simulink model "SecRwLtStFwdBkwdTrgtPosSelc"  (R2018b)
settings: Solver=FixedStepDiscrete  StartTime=0.0  StopTime=10.0  FixedStep=0.01  RelTol=1e-3
undefined symbols (not defined in the file or in its folder): KeSMSw4SAcsMd21SecRwLtStFrwdBkwdPos_Val, KeSMSw4SAcsMd21SecRwLtStFrwdBkwdPosMax_Val, KeSMSw4SAcsMd21SecRwLtStFrwdBkwdPosMin_Val, KeSMSw4SAcsMd22SecRwLtStFrwdBkwdPos_Val, KeSMSw4SAcsMd22SecRwLtStFrwdBkwdPosMax_Val, KeSMSw4SAcsMd22SecRwLtStFrwdBkwdPosMin_Val, KeSMSw4SAcsMd25SecRwLtStFrwdBkwdPos_Val, KeSMSw4SAcsMd25SecRwLtStFrwdBkwdPosMax_Val, KeSMSw4SAcsMd25SecRwLtStFrwdBkwdPosMin_Val, KeSMSw4SAcsMd26SecRwLtStFrwdBkwdPos_Val, KeSMSw4SAcsMd26SecRwLtStFrwdBkwdPosMax_Val, KeSMSw4SAcsMd26SecRwLtStFrwdBkwdPosMin_Val, KeSMSw4SLegrstOpenMdSecRwLtStFrwdBkwdPos_Val, KeSMSw4SLegrstOpenMdSecRwLtStFrwdBkwdPosMax_Val, KeSMSw4SLegrstOpenMdSecRwLtStFrwdBkwdPosMin_Val, KeSMSw4SLyingMDSecRwLtStFrwdBkwdPos_Val, KeSMSw4SLyingMDSecRwLtStFrwdBkwdPosMax_Val, KeSMSw4SLyingMDSecRwLtStFrwdBkwdPosMin_Val, KeSMSw4SVIPMDSecRwLtStFrwdBkwdPos_Val, KeSMSw4SVIPMDSecRwLtStFrwdBkwdPosMax_Val, KeSMSw4SVIPMDSecRwLtStFrwdBkwdPosMin_Val, KeSMSw6sAcsEntrySecRwLtStFrwdBkwdPos_Val, KeSMSw6sAcsEntrySecRwLtStFrwdBkwdPosMax_Val, KeSMSw6sAcsEntrySecRwLtStFrwdBkwdPosMin_Val, KeSMSw6sAcsExtSecRwLtStFrwdBkwdPos_Val, KeSMSw6sAcsExtSecRwLtStFrwdBkwdPosMax_Val, KeSMSw6sAcsExtSecRwLtStFrwdBkwdPosMin_Val, KeSMSw6sFamilyMdSecRwLtStFrwdBkwdPos_Val, KeSMSw6sFamilyMdSecRwLtStFrwdBkwdPosMax_Val, KeSMSw6sFamilyMdSecRwLtStFrwdBkwdPosMin_Val, KeSMSw6sFamilyRMdSecRwLtStFrwdBkwdPos_Val, KeSMSw6sFamilyRMdSecRwLtStFrwdBkwdPosMax_Val, KeSMSw6sFamilyRMdSecRwLtStFrwdBkwdPosMin_Val, KeSMSw6sVIPSecRwLtStFrwdBkwdPos_Val, KeSMSw6sVIPSecRwLtStFrwdBkwdPosMax_Val, KeSMSw6sVIPSecRwLtStFrwdBkwdPosMin_Val, KeSMSwAcsEntrySecRwLtStFrwdBkwdPos_Val, KeSMSwAcsEntrySecRwLtStFrwdBkwdPosMax_Val, KeSMSwAcsEntrySecRwLtStFrwdBkwdPosMin_Val, KeSMSwAcsExtSecRwLtStFrwdBkwdPos_Val, KeSMSwAcsExtSecRwLtStFrwdBkwdPosMax_Val, KeSMSwAcsExtSecRwLtStFrwdBkwdPosMin_Val, KeSMSwAcsMd8SecRwLtStFrwdBkwdPos_Val, KeSMSwAcsMd8SecRwLtStFrwdBkwdPosMax_Val, KeSMSwAcsMd8SecRwLtStFrwdBkwdPosMin_Val, KeSMSwFamilyMdSecRwLtStFrwdBkwdPos_Val, KeSMSwFamilyMdSecRwLtStFrwdBkwdPosMax_Val, KeSMSwFamilyMdSecRwLtStFrwdBkwdPosMin_Val, KeSMSwFamilyRMdSecRwLtStFrwdBkwdPos_Val, KeSMSwFamilyRMdSecRwLtStFrwdBkwdPosMax_Val, KeSMSwFamilyRMdSecRwLtStFrwdBkwdPosMin_Val, KeSMSwVIPSecRwLtStFrwdBkwdPos_Val, KeSMSwVIPSecRwLtStFrwdBkwdPosMax_Val, KeSMSwVIPSecRwLtStFrwdBkwdPosMin_Val
libraries: TrgtPosSelcLib x15
settings Model: Creator=sn2xws  LastModifiedBy=sn2xws
settings Model: ModifiedHistory=|
  | 2023.8.1 V2.0.0 CR401790 增加模式21-26
  | 2023.11.16 V2.3.0 Issue 566045 全躺，vip，腿托打开增加前后位置
  | 2024.7.8 V3.0.0 557模式流程V1.9
settings DataIOCC: SaveFormat=StructureWithTime
settings OptimizationCC: DefaultParameterBehavior=Inlined  EnhancedBackFolding=on  PassReuseOutputArgsAs=Individual arguments  ZeroExternalMemoryAtStartup=off  ZeroInternalMemoryAtStartup=off  OptimizeBlockOrder=speed  DifferentSizesBufferReuse=on  OptimizationCustomize=off
settings DebuggingCC: ParameterTunabilityLossMsg=error
settings HardwareCC: ProdBitPerPointer=32  ProdBitPerSizeT=32  ProdBitPerPtrDiffT=32  ProdLargestAtomicFloat=None  ProdWordSize=32  ProdHWDeviceType=Renesas->RH850
settings ModelReferenceCC: ModelReferenceNumInstancesAllowed=Single
settings SFSimCC: MATLABDynamicMemAlloc=off
settings RTWCC: SystemTargetFile=autosar.tlc  GenCodeOnly=on  TemplateMakefile=ert_default_tmf  Description=AUTOSAR  GenerateReport=on  IncludeHyperlinkInReport=on  LaunchReport=on  GenerateTraceInfo=on  GenerateTraceReport=on  GenerateTraceReportSl=on  GenerateTraceReportSf=on  GenerateTraceReportEml=on  GenerateCodeMetricsReport=on
settings CodeAppCC: ForceParamTrailComments=on  IgnoreCustomStorageClasses=off  OperatorAnnotations=on  SimulinkDataObjDesc=on  SFDataObjDesc=on  InsertBlockDesc=on
settings STFCustomTargetCC: TargetLangStandard=C99 (ISO)  MultiwordLength=256  ParMdlRefBuildCompliant=on  CompOptLevelCompliant=on  IncludeMdlTerminateFcn=off  CombineOutputUpdateFcns=on  SuppressErrorStatus=on  ERTCustomFileBanners=on  SupportNonFinite=off  SupportComplex=off  SupportContinuousTime=off  SupportNonInlinedSFcns=off  RemoveResetFunc=on  MATLABClassNameForMDSCustomization=Simulink.SoftwareTarget.ERTCustomization  AutosarCompliant=on  UseToolchainInfoCompliant=on  LookupTableObjectStructAxisOrder=2,1,3,4,...  LUTObjectStructOrderEvenSpacing=Size,Table,Breakpoints  SystemTargetFile=autosar.tlc
settings ERTTargetCC: TargetLangStandard=C99 (ISO)  ConcurrentExecutionCompliant=off  IncludeMdlTerminateFcn=off  SuppressErrorStatus=on  SupportNonFinite=off  SupportComplex=off  ModelStepFunctionPrototypeControlCompliant=off  CPPClassGenCompliant=off  AutosarCompliant=on  LookupTableObjectStructAxisOrder=2,1,3,4,...  LUTObjectStructOrderEvenSpacing=Size,Table,Breakpoints  InlinedParameterPlacement=NonHierarchical  ERTCustomFileTemplate=example_file_process.tlc  ERTFilePackagingFormat=Compact

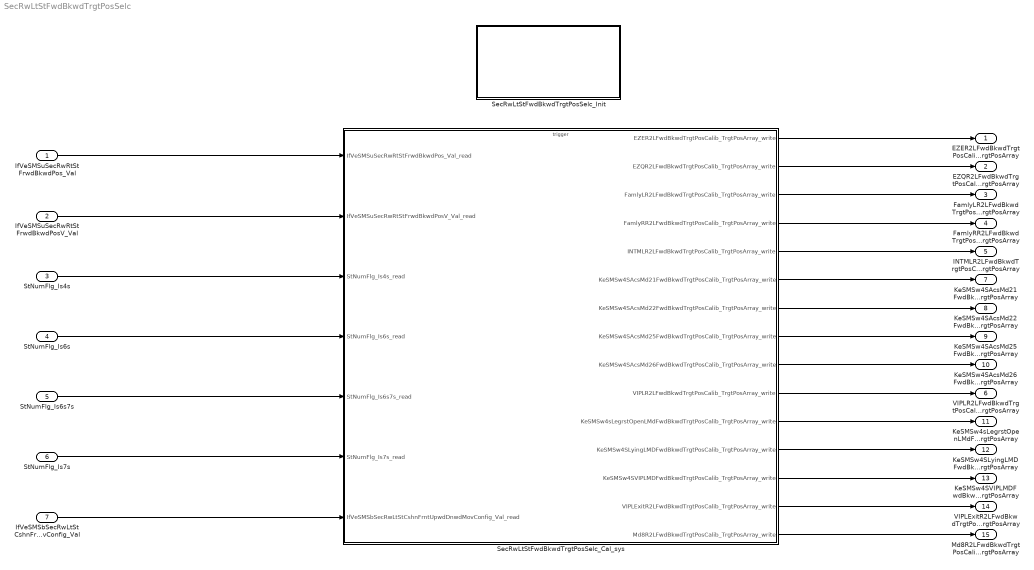
== system SecRwLtStFwdBkwdTrgtPosSelc ==
  IfVeSMSuSecRwRtStFrwdBkwdPos_Val : Inport  OutDataTypeStr=uint16  PortDimensions=1
  IfVeSMSuSecRwRtStFrwdBkwdPosV_Val : Inport  Port=2  OutDataTypeStr=boolean  PortDimensions=1
  StNumFlg_Is4s : Inport  Port=3  OutDataTypeStr=boolean  PortDimensions=1
  StNumFlg_Is6s : Inport  Port=4  OutDataTypeStr=boolean  PortDimensions=1
  StNumFlg_Is6s7s : Inport  Port=5  OutDataTypeStr=boolean  PortDimensions=1
  StNumFlg_Is7s : Inport  Port=6  OutDataTypeStr=boolean  PortDimensions=1
  IfVeSMSbSecRwLtStCshnFrntUpwdDnwdMovConfig_Val : Inport  Port=7  OutDataTypeStr=boolean  PortDimensions=1
  SecRwLtStFwdBkwdTrgtPosSelc_Cal_sys : Subsystem
  SecRwLtStFwdBkwdTrgtPosSelc_Init : Subsystem
  EZER2LFwdBkwdTrgtPosCalib_TrgtPosArray : Outport  Description=|  OutDataTypeStr=uint16  PortDimensions=3
      | 0:Pos
      | 1:Max
      | 2:Min
  EZQR2LFwdBkwdTrgtPosCalib_TrgtPosArray : Outport  Description=|  Port=2  OutDataTypeStr=uint16  PortDimensions=3
      | 0:Pos
      | 1:Max
      | 2:Min
  FamlyLR2LFwdBkwdTrgtPosCalib_TrgtPosArray : Outport  Description=|  Port=3  OutDataTypeStr=uint16  PortDimensions=3
      | 0:Pos
      | 1:Max
      | 2:Min
  FamlyRR2LFwdBkwdTrgtPosCalib_TrgtPosArray : Outport  Description=|  Port=4  OutDataTypeStr=uint16  PortDimensions=3
      | 0:Pos
      | 1:Max
      | 2:Min
  INTMLR2LFwdBkwdTrgtPosCalib_TrgtPosArray : Outport  Description=|  Port=5  OutDataTypeStr=uint16  PortDimensions=3
      | 0:Pos
      | 1:Max
      | 2:Min
  VIPLR2LFwdBkwdTrgtPosCalib_TrgtPosArray : Outport  Description=|  Port=6  OutDataTypeStr=uint16  PortDimensions=3
      | 0:Pos
      | 1:Max
      | 2:Min
  KeSMSw4SAcsMd21FwdBkwdTrgtPosCalib_TrgtPosArray : Outport  Description=|  Port=7  OutDataTypeStr=uint16  PortDimensions=3
      | 0:Pos
      | 1:Max
      | 2:Min
  KeSMSw4SAcsMd22FwdBkwdTrgtPosCalib_TrgtPosArray : Outport  Description=|  Port=8  OutDataTypeStr=uint16  PortDimensions=3
      | 0:Pos
      | 1:Max
      | 2:Min
  KeSMSw4SAcsMd25FwdBkwdTrgtPosCalib_TrgtPosArray : Outport  Description=|  Port=9  OutDataTypeStr=uint16  PortDimensions=3
      | 0:Pos
      | 1:Max
      | 2:Min
  KeSMSw4SAcsMd26FwdBkwdTrgtPosCalib_TrgtPosArray : Outport  Description=|  Port=10  OutDataTypeStr=uint16  PortDimensions=3
      | 0:Pos
      | 1:Max
      | 2:Min
  KeSMSw4sLegrstOpenLMdFwdBkwdTrgtPosCalib_TrgtPosArray : Outport  Description=|  Port=11  OutDataTypeStr=uint16  PortDimensions=3
      | 0:Pos
      | 1:Max
      | 2:Min
  KeSMSw4SLyingLMDFwdBkwdTrgtPosCalib_TrgtPosArray : Outport  Description=|  Port=12  OutDataTypeStr=uint16  PortDimensions=3
      | 0:Pos
      | 1:Max
      | 2:Min
  KeSMSw4SVIPLMDFwdBkwdTrgtPosCalib_TrgtPosArray : Outport  Description=|  Port=13  OutDataTypeStr=uint16  PortDimensions=3
      | 0:Pos
      | 1:Max
      | 2:Min
  VIPLExitR2LFwdBkwdTrgtPosCalib_TrgtPosArray : Outport  Description=|  Port=14  OutDataTypeStr=uint16  PortDimensions=3
      | 0:Pos
      | 1:Max
      | 2:Min
  Md8R2LFwdBkwdTrgtPosCalib_TrgtPosArray : Outport  Description=|  Port=15  OutDataTypeStr=uint16  PortDimensions=3
      | 0:Pos
      | 1:Max
      | 2:Min
  wires:
  IfVeSMSuSecRwRtStFrwdBkwdPos_Val/1 -> SecRwLtStFwdBkwdTrgtPosSelc_Cal_sys/1(IfVeSMSuSecRwRtStFrwdBkwdPos_Val_read)
  IfVeSMSuSecRwRtStFrwdBkwdPosV_Val/1 -> SecRwLtStFwdBkwdTrgtPosSelc_Cal_sys/2(IfVeSMSuSecRwRtStFrwdBkwdPosV_Val_read)
  StNumFlg_Is4s/1 -> SecRwLtStFwdBkwdTrgtPosSelc_Cal_sys/3(StNumFlg_Is4s_read)
  StNumFlg_Is6s/1 -> SecRwLtStFwdBkwdTrgtPosSelc_Cal_sys/4(StNumFlg_Is6s_read)
  StNumFlg_Is6s7s/1 -> SecRwLtStFwdBkwdTrgtPosSelc_Cal_sys/5(StNumFlg_Is6s7s_read)
  StNumFlg_Is7s/1 -> SecRwLtStFwdBkwdTrgtPosSelc_Cal_sys/6(StNumFlg_Is7s_read)
  SecRwLtStFwdBkwdTrgtPosSelc_Cal_sys/1(EZER2LFwdBkwdTrgtPosCalib_TrgtPosArray_write) -> EZER2LFwdBkwdTrgtPosCalib_TrgtPosArray/1
  SecRwLtStFwdBkwdTrgtPosSelc_Cal_sys/2(EZQR2LFwdBkwdTrgtPosCalib_TrgtPosArray_write) -> EZQR2LFwdBkwdTrgtPosCalib_TrgtPosArray/1
  SecRwLtStFwdBkwdTrgtPosSelc_Cal_sys/3(FamlyLR2LFwdBkwdTrgtPosCalib_TrgtPosArray_write) -> FamlyLR2LFwdBkwdTrgtPosCalib_TrgtPosArray/1
  SecRwLtStFwdBkwdTrgtPosSelc_Cal_sys/4(FamlyRR2LFwdBkwdTrgtPosCalib_TrgtPosArray_write) -> FamlyRR2LFwdBkwdTrgtPosCalib_TrgtPosArray/1
  SecRwLtStFwdBkwdTrgtPosSelc_Cal_sys/5(INTMLR2LFwdBkwdTrgtPosCalib_TrgtPosArray_write) -> INTMLR2LFwdBkwdTrgtPosCalib_TrgtPosArray/1
  SecRwLtStFwdBkwdTrgtPosSelc_Cal_sys/10(VIPLR2LFwdBkwdTrgtPosCalib_TrgtPosArray_write) -> VIPLR2LFwdBkwdTrgtPosCalib_TrgtPosArray/1
  SecRwLtStFwdBkwdTrgtPosSelc_Cal_sys/6(KeSMSw4SAcsMd21FwdBkwdTrgtPosCalib_TrgtPosArray_write) -> KeSMSw4SAcsMd21FwdBkwdTrgtPosCalib_TrgtPosArray/1
  SecRwLtStFwdBkwdTrgtPosSelc_Cal_sys/7(KeSMSw4SAcsMd22FwdBkwdTrgtPosCalib_TrgtPosArray_write) -> KeSMSw4SAcsMd22FwdBkwdTrgtPosCalib_TrgtPosArray/1
  SecRwLtStFwdBkwdTrgtPosSelc_Cal_sys/8(KeSMSw4SAcsMd25FwdBkwdTrgtPosCalib_TrgtPosArray_write) -> KeSMSw4SAcsMd25FwdBkwdTrgtPosCalib_TrgtPosArray/1
  SecRwLtStFwdBkwdTrgtPosSelc_Cal_sys/9(KeSMSw4SAcsMd26FwdBkwdTrgtPosCalib_TrgtPosArray_write) -> KeSMSw4SAcsMd26FwdBkwdTrgtPosCalib_TrgtPosArray/1
  SecRwLtStFwdBkwdTrgtPosSelc_Cal_sys/11(KeSMSw4sLegrstOpenLMdFwdBkwdTrgtPosCalib_TrgtPosArray_write) -> KeSMSw4sLegrstOpenLMdFwdBkwdTrgtPosCalib_TrgtPosArray/1
  SecRwLtStFwdBkwdTrgtPosSelc_Cal_sys/12(KeSMSw4SLyingLMDFwdBkwdTrgtPosCalib_TrgtPosArray_write) -> KeSMSw4SLyingLMDFwdBkwdTrgtPosCalib_TrgtPosArray/1
  SecRwLtStFwdBkwdTrgtPosSelc_Cal_sys/13(KeSMSw4SVIPLMDFwdBkwdTrgtPosCalib_TrgtPosArray_write) -> KeSMSw4SVIPLMDFwdBkwdTrgtPosCalib_TrgtPosArray/1
  IfVeSMSbSecRwLtStCshnFrntUpwdDnwdMovConfig_Val/1 -> SecRwLtStFwdBkwdTrgtPosSelc_Cal_sys/7(IfVeSMSbSecRwLtStCshnFrntUpwdDnwdMovConfig_Val_read)
  SecRwLtStFwdBkwdTrgtPosSelc_Cal_sys/14(VIPLExitR2LFwdBkwdTrgtPosCalib_TrgtPosArray_write) -> VIPLExitR2LFwdBkwdTrgtPosCalib_TrgtPosArray/1
  SecRwLtStFwdBkwdTrgtPosSelc_Cal_sys/15(Md8R2LFwdBkwdTrgtPosCalib_TrgtPosArray_write) -> Md8R2LFwdBkwdTrgtPosCalib_TrgtPosArray/1

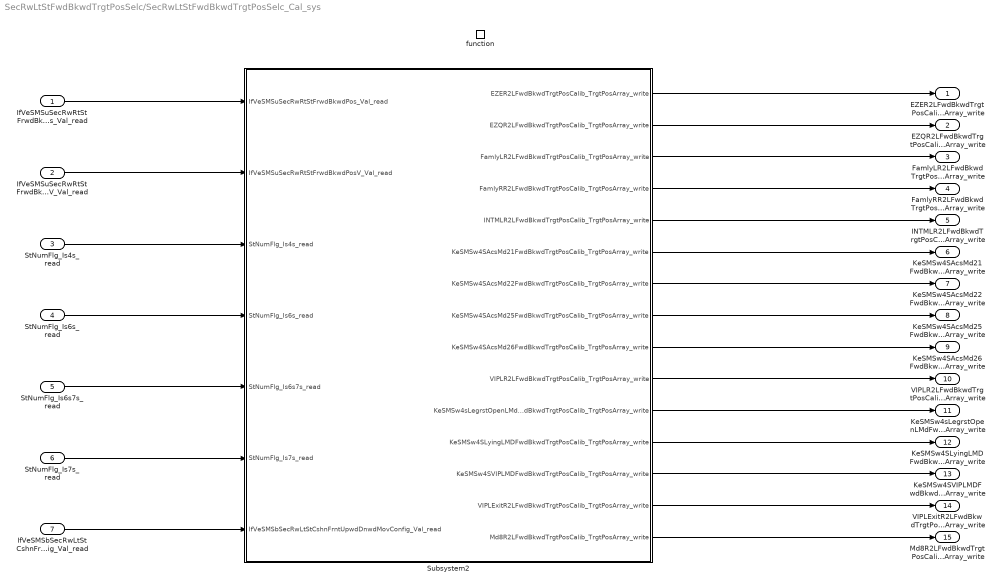
== system SecRwLtStFwdBkwdTrgtPosSelc/SecRwLtStFwdBkwdTrgtPosSelc_Cal_sys ==
  IfVeSMSuSecRwRtStFrwdBkwdPos_Val_read : Inport
  IfVeSMSuSecRwRtStFrwdBkwdPosV_Val_read : Inport  Port=2
  StNumFlg_Is4s_read : Inport  Port=3
  StNumFlg_Is6s_read : Inport  Port=4
  StNumFlg_Is6s7s_read : Inport  Port=5
  StNumFlg_Is7s_read : Inport  Port=6
  IfVeSMSbSecRwLtStCshnFrntUpwdDnwdMovConfig_Val_read : Inport  Port=7
  function : TriggerPort  TriggerType=function-call  IsSimulinkFunction=on  FunctionName=SecRwLtStFwdBkwdTrgtPosSelc_Cal  VariantControl=(inherit)
  Subsystem2 : Subsystem
  EZER2LFwdBkwdTrgtPosCalib_TrgtPosArray_write : Outport
      settings: EnsureOutportIsVirtual=on
  EZQR2LFwdBkwdTrgtPosCalib_TrgtPosArray_write : Outport  Port=2
      settings: EnsureOutportIsVirtual=on
  FamlyLR2LFwdBkwdTrgtPosCalib_TrgtPosArray_write : Outport  Port=3
      settings: EnsureOutportIsVirtual=on
  FamlyRR2LFwdBkwdTrgtPosCalib_TrgtPosArray_write : Outport  Port=4
      settings: EnsureOutportIsVirtual=on
  INTMLR2LFwdBkwdTrgtPosCalib_TrgtPosArray_write : Outport  Port=5
      settings: EnsureOutportIsVirtual=on
  KeSMSw4SAcsMd21FwdBkwdTrgtPosCalib_TrgtPosArray_write : Outport  Port=6
      settings: EnsureOutportIsVirtual=on
  KeSMSw4SAcsMd22FwdBkwdTrgtPosCalib_TrgtPosArray_write : Outport  Port=7
      settings: EnsureOutportIsVirtual=on
  KeSMSw4SAcsMd25FwdBkwdTrgtPosCalib_TrgtPosArray_write : Outport  Port=8
      settings: EnsureOutportIsVirtual=on
  KeSMSw4SAcsMd26FwdBkwdTrgtPosCalib_TrgtPosArray_write : Outport  Port=9
      settings: EnsureOutportIsVirtual=on
  VIPLR2LFwdBkwdTrgtPosCalib_TrgtPosArray_write : Outport  Port=10
      settings: EnsureOutportIsVirtual=on
  KeSMSw4sLegrstOpenLMdFwdBkwdTrgtPosCalib_TrgtPosArray_write : Outport  Port=11
      settings: EnsureOutportIsVirtual=on
  KeSMSw4SLyingLMDFwdBkwdTrgtPosCalib_TrgtPosArray_write : Outport  Port=12
      settings: EnsureOutportIsVirtual=on
  KeSMSw4SVIPLMDFwdBkwdTrgtPosCalib_TrgtPosArray_write : Outport  Port=13
      settings: EnsureOutportIsVirtual=on
  VIPLExitR2LFwdBkwdTrgtPosCalib_TrgtPosArray_write : Outport  Port=14
      settings: EnsureOutportIsVirtual=on
  Md8R2LFwdBkwdTrgtPosCalib_TrgtPosArray_write : Outport  Port=15
      settings: EnsureOutportIsVirtual=on
  wires:
  Subsystem2/9(KeSMSw4SAcsMd26FwdBkwdTrgtPosCalib_TrgtPosArray_write) -> KeSMSw4SAcsMd26FwdBkwdTrgtPosCalib_TrgtPosArray_write/1
  Subsystem2/10(VIPLR2LFwdBkwdTrgtPosCalib_TrgtPosArray_write) -> VIPLR2LFwdBkwdTrgtPosCalib_TrgtPosArray_write/1
  Subsystem2/6(KeSMSw4SAcsMd21FwdBkwdTrgtPosCalib_TrgtPosArray_write) -> KeSMSw4SAcsMd21FwdBkwdTrgtPosCalib_TrgtPosArray_write/1
  Subsystem2/7(KeSMSw4SAcsMd22FwdBkwdTrgtPosCalib_TrgtPosArray_write) -> KeSMSw4SAcsMd22FwdBkwdTrgtPosCalib_TrgtPosArray_write/1
  Subsystem2/8(KeSMSw4SAcsMd25FwdBkwdTrgtPosCalib_TrgtPosArray_write) -> KeSMSw4SAcsMd25FwdBkwdTrgtPosCalib_TrgtPosArray_write/1
  Subsystem2/4(FamlyRR2LFwdBkwdTrgtPosCalib_TrgtPosArray_write) -> FamlyRR2LFwdBkwdTrgtPosCalib_TrgtPosArray_write/1
  Subsystem2/5(INTMLR2LFwdBkwdTrgtPosCalib_TrgtPosArray_write) -> INTMLR2LFwdBkwdTrgtPosCalib_TrgtPosArray_write/1
  Subsystem2/1(EZER2LFwdBkwdTrgtPosCalib_TrgtPosArray_write) -> EZER2LFwdBkwdTrgtPosCalib_TrgtPosArray_write/1
  Subsystem2/2(EZQR2LFwdBkwdTrgtPosCalib_TrgtPosArray_write) -> EZQR2LFwdBkwdTrgtPosCalib_TrgtPosArray_write/1
  Subsystem2/3(FamlyLR2LFwdBkwdTrgtPosCalib_TrgtPosArray_write) -> FamlyLR2LFwdBkwdTrgtPosCalib_TrgtPosArray_write/1
  IfVeSMSuSecRwRtStFrwdBkwdPos_Val_read/1 -> Subsystem2/1(IfVeSMSuSecRwRtStFrwdBkwdPos_Val_read)
  IfVeSMSuSecRwRtStFrwdBkwdPosV_Val_read/1 -> Subsystem2/2(IfVeSMSuSecRwRtStFrwdBkwdPosV_Val_read)
  StNumFlg_Is4s_read/1 -> Subsystem2/3(StNumFlg_Is4s_read)
  StNumFlg_Is6s_read/1 -> Subsystem2/4(StNumFlg_Is6s_read)
  StNumFlg_Is6s7s_read/1 -> Subsystem2/5(StNumFlg_Is6s7s_read)
  StNumFlg_Is7s_read/1 -> Subsystem2/6(StNumFlg_Is7s_read)
  Subsystem2/11(KeSMSw4sLegrstOpenLMdFwdBkwdTrgtPosCalib_TrgtPosArray_write) -> KeSMSw4sLegrstOpenLMdFwdBkwdTrgtPosCalib_TrgtPosArray_write/1
  Subsystem2/12(KeSMSw4SLyingLMDFwdBkwdTrgtPosCalib_TrgtPosArray_write) -> KeSMSw4SLyingLMDFwdBkwdTrgtPosCalib_TrgtPosArray_write/1
  Subsystem2/13(KeSMSw4SVIPLMDFwdBkwdTrgtPosCalib_TrgtPosArray_write) -> KeSMSw4SVIPLMDFwdBkwdTrgtPosCalib_TrgtPosArray_write/1
  Subsystem2/14(VIPLExitR2LFwdBkwdTrgtPosCalib_TrgtPosArray_write) -> VIPLExitR2LFwdBkwdTrgtPosCalib_TrgtPosArray_write/1
  IfVeSMSbSecRwLtStCshnFrntUpwdDnwdMovConfig_Val_read/1 -> Subsystem2/7(IfVeSMSbSecRwLtStCshnFrntUpwdDnwdMovConfig_Val_read)
  Subsystem2/15(Md8R2LFwdBkwdTrgtPosCalib_TrgtPosArray_write) -> Md8R2LFwdBkwdTrgtPosCalib_TrgtPosArray_write/1

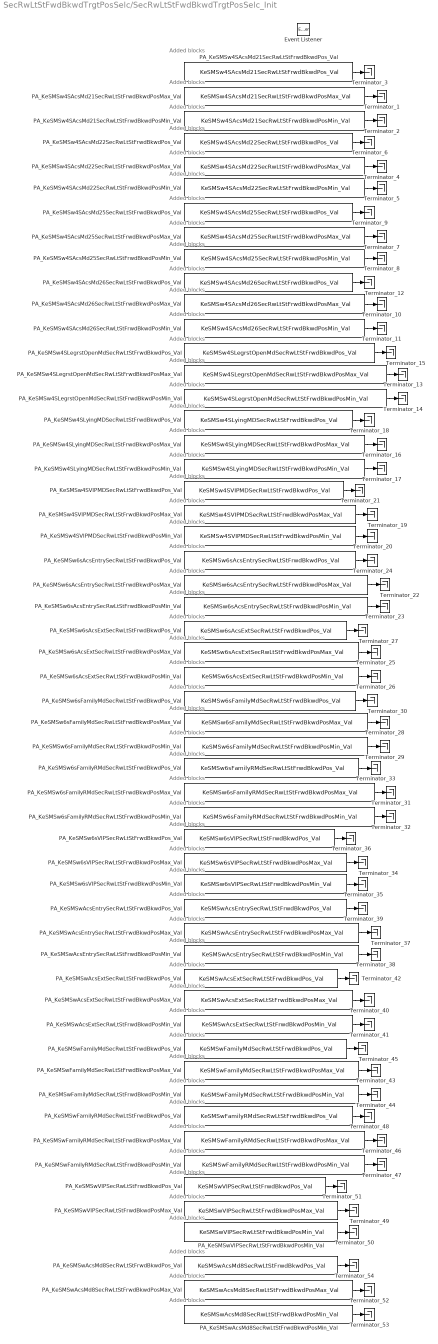
== system SecRwLtStFwdBkwdTrgtPosSelc/SecRwLtStFwdBkwdTrgtPosSelc_Init ==
  note: Added blocks
  note: Added blocks
  note: Added blocks
  note: Added blocks
  note: Added blocks
  note: Added blocks
  note: Added blocks
  note: Added blocks
  note: Added blocks
  note: Added blocks
  note: Added blocks
  note: Added blocks
  note: Added blocks
  note: Added blocks
  note: Added blocks
  note: Added blocks
  note: Added blocks
  note: Added blocks
  note: Added blocks
  note: Added blocks
  note: Added blocks
  note: Added blocks
  note: Added blocks
  note: Added blocks
  note: Added blocks
  note: Added blocks
  note: Added blocks
  note: Added blocks
  note: Added blocks
  note: Added blocks
  note: Added blocks
  note: Added blocks
  note: Added blocks
  note: Added blocks
  note: Added blocks
  note: Added blocks
  note: Added blocks
  note: Added blocks
  note: Added blocks
  note: Added blocks
  note: Added blocks
  note: Added blocks
  note: Added blocks
  note: Added blocks
  note: Added blocks
  note: Added blocks
  note: Added blocks
  note: Added blocks
  note: Added blocks
  note: Added blocks
  note: Added blocks
  note: Added blocks
  note: Added blocks
  note: Added blocks
  Event Listener : EventListener  EventName=reset
  PA_KeSMSw4SAcsMd21SecRwLtStFrwdBkwdPosMax_Val : Constant  Value=KeSMSw4SAcsMd21SecRwLtStFrwdBkwdPosMax_Val
  PA_KeSMSw4SAcsMd21SecRwLtStFrwdBkwdPosMin_Val : Constant  Value=KeSMSw4SAcsMd21SecRwLtStFrwdBkwdPosMin_Val
  PA_KeSMSw4SAcsMd21SecRwLtStFrwdBkwdPos_Val : Constant  Value=KeSMSw4SAcsMd21SecRwLtStFrwdBkwdPos_Val
  PA_KeSMSw4SAcsMd22SecRwLtStFrwdBkwdPosMax_Val : Constant  Value=KeSMSw4SAcsMd22SecRwLtStFrwdBkwdPosMax_Val
  PA_KeSMSw4SAcsMd22SecRwLtStFrwdBkwdPosMin_Val : Constant  Value=KeSMSw4SAcsMd22SecRwLtStFrwdBkwdPosMin_Val
  PA_KeSMSw4SAcsMd22SecRwLtStFrwdBkwdPos_Val : Constant  Value=KeSMSw4SAcsMd22SecRwLtStFrwdBkwdPos_Val
  PA_KeSMSw4SAcsMd25SecRwLtStFrwdBkwdPosMax_Val : Constant  Value=KeSMSw4SAcsMd25SecRwLtStFrwdBkwdPosMax_Val
  PA_KeSMSw4SAcsMd25SecRwLtStFrwdBkwdPosMin_Val : Constant  Value=KeSMSw4SAcsMd25SecRwLtStFrwdBkwdPosMin_Val
  PA_KeSMSw4SAcsMd25SecRwLtStFrwdBkwdPos_Val : Constant  Value=KeSMSw4SAcsMd25SecRwLtStFrwdBkwdPos_Val
  PA_KeSMSw4SAcsMd26SecRwLtStFrwdBkwdPosMax_Val : Constant  Value=KeSMSw4SAcsMd26SecRwLtStFrwdBkwdPosMax_Val
  PA_KeSMSw4SAcsMd26SecRwLtStFrwdBkwdPosMin_Val : Constant  Value=KeSMSw4SAcsMd26SecRwLtStFrwdBkwdPosMin_Val
  PA_KeSMSw4SAcsMd26SecRwLtStFrwdBkwdPos_Val : Constant  Value=KeSMSw4SAcsMd26SecRwLtStFrwdBkwdPos_Val
  PA_KeSMSw4SLegrstOpenMdSecRwLtStFrwdBkwdPosMax_Val : Constant  Value=KeSMSw4SLegrstOpenMdSecRwLtStFrwdBkwdPosMax_Val
  PA_KeSMSw4SLegrstOpenMdSecRwLtStFrwdBkwdPosMin_Val : Constant  Value=KeSMSw4SLegrstOpenMdSecRwLtStFrwdBkwdPosMin_Val
  PA_KeSMSw4SLegrstOpenMdSecRwLtStFrwdBkwdPos_Val : Constant  Value=KeSMSw4SLegrstOpenMdSecRwLtStFrwdBkwdPos_Val
  PA_KeSMSw4SLyingMDSecRwLtStFrwdBkwdPosMax_Val : Constant  Value=KeSMSw4SLyingMDSecRwLtStFrwdBkwdPosMax_Val
  PA_KeSMSw4SLyingMDSecRwLtStFrwdBkwdPosMin_Val : Constant  Value=KeSMSw4SLyingMDSecRwLtStFrwdBkwdPosMin_Val
  PA_KeSMSw4SLyingMDSecRwLtStFrwdBkwdPos_Val : Constant  Value=KeSMSw4SLyingMDSecRwLtStFrwdBkwdPos_Val
  PA_KeSMSw4SVIPMDSecRwLtStFrwdBkwdPosMax_Val : Constant  Value=KeSMSw4SVIPMDSecRwLtStFrwdBkwdPosMax_Val
  PA_KeSMSw4SVIPMDSecRwLtStFrwdBkwdPosMin_Val : Constant  Value=KeSMSw4SVIPMDSecRwLtStFrwdBkwdPosMin_Val
  PA_KeSMSw4SVIPMDSecRwLtStFrwdBkwdPos_Val : Constant  Value=KeSMSw4SVIPMDSecRwLtStFrwdBkwdPos_Val
  PA_KeSMSw6sAcsEntrySecRwLtStFrwdBkwdPosMax_Val : Constant  Value=KeSMSw6sAcsEntrySecRwLtStFrwdBkwdPosMax_Val
  PA_KeSMSw6sAcsEntrySecRwLtStFrwdBkwdPosMin_Val : Constant  Value=KeSMSw6sAcsEntrySecRwLtStFrwdBkwdPosMin_Val
  PA_KeSMSw6sAcsEntrySecRwLtStFrwdBkwdPos_Val : Constant  Value=KeSMSw6sAcsEntrySecRwLtStFrwdBkwdPos_Val
  PA_KeSMSw6sAcsExtSecRwLtStFrwdBkwdPosMax_Val : Constant  Value=KeSMSw6sAcsExtSecRwLtStFrwdBkwdPosMax_Val
  PA_KeSMSw6sAcsExtSecRwLtStFrwdBkwdPosMin_Val : Constant  Value=KeSMSw6sAcsExtSecRwLtStFrwdBkwdPosMin_Val
  PA_KeSMSw6sAcsExtSecRwLtStFrwdBkwdPos_Val : Constant  Value=KeSMSw6sAcsExtSecRwLtStFrwdBkwdPos_Val
  PA_KeSMSw6sFamilyMdSecRwLtStFrwdBkwdPosMax_Val : Constant  Value=KeSMSw6sFamilyMdSecRwLtStFrwdBkwdPosMax_Val
  PA_KeSMSw6sFamilyMdSecRwLtStFrwdBkwdPosMin_Val : Constant  Value=KeSMSw6sFamilyMdSecRwLtStFrwdBkwdPosMin_Val
  PA_KeSMSw6sFamilyMdSecRwLtStFrwdBkwdPos_Val : Constant  Value=KeSMSw6sFamilyMdSecRwLtStFrwdBkwdPos_Val
  PA_KeSMSw6sFamilyRMdSecRwLtStFrwdBkwdPosMax_Val : Constant  Value=KeSMSw6sFamilyRMdSecRwLtStFrwdBkwdPosMax_Val
  PA_KeSMSw6sFamilyRMdSecRwLtStFrwdBkwdPosMin_Val : Constant  Value=KeSMSw6sFamilyRMdSecRwLtStFrwdBkwdPosMin_Val
  PA_KeSMSw6sFamilyRMdSecRwLtStFrwdBkwdPos_Val : Constant  Value=KeSMSw6sFamilyRMdSecRwLtStFrwdBkwdPos_Val
  PA_KeSMSw6sVIPSecRwLtStFrwdBkwdPosMax_Val : Constant  Value=KeSMSw6sVIPSecRwLtStFrwdBkwdPosMax_Val
  PA_KeSMSw6sVIPSecRwLtStFrwdBkwdPosMin_Val : Constant  Value=KeSMSw6sVIPSecRwLtStFrwdBkwdPosMin_Val
  PA_KeSMSw6sVIPSecRwLtStFrwdBkwdPos_Val : Constant  Value=KeSMSw6sVIPSecRwLtStFrwdBkwdPos_Val
  PA_KeSMSwAcsEntrySecRwLtStFrwdBkwdPosMax_Val : Constant  Value=KeSMSwAcsEntrySecRwLtStFrwdBkwdPosMax_Val
  PA_KeSMSwAcsEntrySecRwLtStFrwdBkwdPosMin_Val : Constant  Value=KeSMSwAcsEntrySecRwLtStFrwdBkwdPosMin_Val
  PA_KeSMSwAcsEntrySecRwLtStFrwdBkwdPos_Val : Constant  Value=KeSMSwAcsEntrySecRwLtStFrwdBkwdPos_Val
  PA_KeSMSwAcsExtSecRwLtStFrwdBkwdPosMax_Val : Constant  Value=KeSMSwAcsExtSecRwLtStFrwdBkwdPosMax_Val
  PA_KeSMSwAcsExtSecRwLtStFrwdBkwdPosMin_Val : Constant  Value=KeSMSwAcsExtSecRwLtStFrwdBkwdPosMin_Val
  PA_KeSMSwAcsExtSecRwLtStFrwdBkwdPos_Val : Constant  Value=KeSMSwAcsExtSecRwLtStFrwdBkwdPos_Val
  PA_KeSMSwAcsMd8SecRwLtStFrwdBkwdPosMax_Val : Constant  Value=KeSMSwAcsMd8SecRwLtStFrwdBkwdPosMax_Val
  PA_KeSMSwAcsMd8SecRwLtStFrwdBkwdPosMin_Val : Constant  Value=KeSMSwAcsMd8SecRwLtStFrwdBkwdPosMin_Val
  PA_KeSMSwAcsMd8SecRwLtStFrwdBkwdPos_Val : Constant  Value=KeSMSwAcsMd8SecRwLtStFrwdBkwdPos_Val
  PA_KeSMSwFamilyMdSecRwLtStFrwdBkwdPosMax_Val : Constant  Value=KeSMSwFamilyMdSecRwLtStFrwdBkwdPosMax_Val
  PA_KeSMSwFamilyMdSecRwLtStFrwdBkwdPosMin_Val : Constant  Value=KeSMSwFamilyMdSecRwLtStFrwdBkwdPosMin_Val
  PA_KeSMSwFamilyMdSecRwLtStFrwdBkwdPos_Val : Constant  Value=KeSMSwFamilyMdSecRwLtStFrwdBkwdPos_Val
  PA_KeSMSwFamilyRMdSecRwLtStFrwdBkwdPosMax_Val : Constant  Value=KeSMSwFamilyRMdSecRwLtStFrwdBkwdPosMax_Val
  PA_KeSMSwFamilyRMdSecRwLtStFrwdBkwdPosMin_Val : Constant  Value=KeSMSwFamilyRMdSecRwLtStFrwdBkwdPosMin_Val
  PA_KeSMSwFamilyRMdSecRwLtStFrwdBkwdPos_Val : Constant  Value=KeSMSwFamilyRMdSecRwLtStFrwdBkwdPos_Val
  PA_KeSMSwVIPSecRwLtStFrwdBkwdPosMax_Val : Constant  Value=KeSMSwVIPSecRwLtStFrwdBkwdPosMax_Val
  PA_KeSMSwVIPSecRwLtStFrwdBkwdPosMin_Val : Constant  Value=KeSMSwVIPSecRwLtStFrwdBkwdPosMin_Val
  PA_KeSMSwVIPSecRwLtStFrwdBkwdPos_Val : Constant  Value=KeSMSwVIPSecRwLtStFrwdBkwdPos_Val
  Terminator_{1..54} (54 alike) : Terminator
  wires:
  PA_KeSMSw4SAcsMd21SecRwLtStFrwdBkwdPosMax_Val/1 -> Terminator_1/1
  PA_KeSMSw4SAcsMd21SecRwLtStFrwdBkwdPosMin_Val/1 -> Terminator_2/1
  PA_KeSMSw4SAcsMd21SecRwLtStFrwdBkwdPos_Val/1 -> Terminator_3/1
  PA_KeSMSw4SAcsMd22SecRwLtStFrwdBkwdPosMax_Val/1 -> Terminator_4/1
  PA_KeSMSw4SAcsMd22SecRwLtStFrwdBkwdPosMin_Val/1 -> Terminator_5/1
  PA_KeSMSw4SAcsMd22SecRwLtStFrwdBkwdPos_Val/1 -> Terminator_6/1
  PA_KeSMSw4SAcsMd25SecRwLtStFrwdBkwdPosMax_Val/1 -> Terminator_7/1
  PA_KeSMSw4SAcsMd25SecRwLtStFrwdBkwdPosMin_Val/1 -> Terminator_8/1
  PA_KeSMSw4SAcsMd25SecRwLtStFrwdBkwdPos_Val/1 -> Terminator_9/1
  PA_KeSMSw4SAcsMd26SecRwLtStFrwdBkwdPosMax_Val/1 -> Terminator_10/1
  PA_KeSMSw4SAcsMd26SecRwLtStFrwdBkwdPosMin_Val/1 -> Terminator_11/1
  PA_KeSMSw4SAcsMd26SecRwLtStFrwdBkwdPos_Val/1 -> Terminator_12/1
  PA_KeSMSw4SLegrstOpenMdSecRwLtStFrwdBkwdPosMax_Val/1 -> Terminator_13/1
  PA_KeSMSw4SLegrstOpenMdSecRwLtStFrwdBkwdPosMin_Val/1 -> Terminator_14/1
  PA_KeSMSw4SLegrstOpenMdSecRwLtStFrwdBkwdPos_Val/1 -> Terminator_15/1
  PA_KeSMSw4SLyingMDSecRwLtStFrwdBkwdPosMax_Val/1 -> Terminator_16/1
  PA_KeSMSw4SLyingMDSecRwLtStFrwdBkwdPosMin_Val/1 -> Terminator_17/1
  PA_KeSMSw4SLyingMDSecRwLtStFrwdBkwdPos_Val/1 -> Terminator_18/1
  PA_KeSMSw4SVIPMDSecRwLtStFrwdBkwdPosMax_Val/1 -> Terminator_19/1
  PA_KeSMSw4SVIPMDSecRwLtStFrwdBkwdPosMin_Val/1 -> Terminator_20/1
  PA_KeSMSw4SVIPMDSecRwLtStFrwdBkwdPos_Val/1 -> Terminator_21/1
  PA_KeSMSw6sAcsEntrySecRwLtStFrwdBkwdPosMax_Val/1 -> Terminator_22/1
  PA_KeSMSw6sAcsEntrySecRwLtStFrwdBkwdPosMin_Val/1 -> Terminator_23/1
  PA_KeSMSw6sAcsEntrySecRwLtStFrwdBkwdPos_Val/1 -> Terminator_24/1
  PA_KeSMSw6sAcsExtSecRwLtStFrwdBkwdPosMax_Val/1 -> Terminator_25/1
  PA_KeSMSw6sAcsExtSecRwLtStFrwdBkwdPosMin_Val/1 -> Terminator_26/1
  PA_KeSMSw6sAcsExtSecRwLtStFrwdBkwdPos_Val/1 -> Terminator_27/1
  PA_KeSMSw6sFamilyMdSecRwLtStFrwdBkwdPosMax_Val/1 -> Terminator_28/1
  PA_KeSMSw6sFamilyMdSecRwLtStFrwdBkwdPosMin_Val/1 -> Terminator_29/1
  PA_KeSMSw6sFamilyMdSecRwLtStFrwdBkwdPos_Val/1 -> Terminator_30/1
  PA_KeSMSw6sFamilyRMdSecRwLtStFrwdBkwdPosMax_Val/1 -> Terminator_31/1
  PA_KeSMSw6sFamilyRMdSecRwLtStFrwdBkwdPosMin_Val/1 -> Terminator_32/1
  PA_KeSMSw6sFamilyRMdSecRwLtStFrwdBkwdPos_Val/1 -> Terminator_33/1
  PA_KeSMSw6sVIPSecRwLtStFrwdBkwdPosMax_Val/1 -> Terminator_34/1
  PA_KeSMSw6sVIPSecRwLtStFrwdBkwdPosMin_Val/1 -> Terminator_35/1
  PA_KeSMSw6sVIPSecRwLtStFrwdBkwdPos_Val/1 -> Terminator_36/1
  PA_KeSMSwAcsEntrySecRwLtStFrwdBkwdPosMax_Val/1 -> Terminator_37/1
  PA_KeSMSwAcsEntrySecRwLtStFrwdBkwdPosMin_Val/1 -> Terminator_38/1
  PA_KeSMSwAcsEntrySecRwLtStFrwdBkwdPos_Val/1 -> Terminator_39/1
  PA_KeSMSwAcsExtSecRwLtStFrwdBkwdPosMax_Val/1 -> Terminator_40/1
  PA_KeSMSwAcsExtSecRwLtStFrwdBkwdPosMin_Val/1 -> Terminator_41/1
  PA_KeSMSwAcsExtSecRwLtStFrwdBkwdPos_Val/1 -> Terminator_42/1
  PA_KeSMSwFamilyMdSecRwLtStFrwdBkwdPosMax_Val/1 -> Terminator_43/1
  PA_KeSMSwFamilyMdSecRwLtStFrwdBkwdPosMin_Val/1 -> Terminator_44/1
  PA_KeSMSwFamilyMdSecRwLtStFrwdBkwdPos_Val/1 -> Terminator_45/1
  PA_KeSMSwFamilyRMdSecRwLtStFrwdBkwdPosMax_Val/1 -> Terminator_46/1
  PA_KeSMSwFamilyRMdSecRwLtStFrwdBkwdPosMin_Val/1 -> Terminator_47/1
  PA_KeSMSwFamilyRMdSecRwLtStFrwdBkwdPos_Val/1 -> Terminator_48/1
  PA_KeSMSwVIPSecRwLtStFrwdBkwdPosMax_Val/1 -> Terminator_49/1
  PA_KeSMSwVIPSecRwLtStFrwdBkwdPosMin_Val/1 -> Terminator_50/1
  PA_KeSMSwVIPSecRwLtStFrwdBkwdPos_Val/1 -> Terminator_51/1
  PA_KeSMSwAcsMd8SecRwLtStFrwdBkwdPosMax_Val/1 -> Terminator_52/1
  PA_KeSMSwAcsMd8SecRwLtStFrwdBkwdPosMin_Val/1 -> Terminator_53/1
  PA_KeSMSwAcsMd8SecRwLtStFrwdBkwdPos_Val/1 -> Terminator_54/1

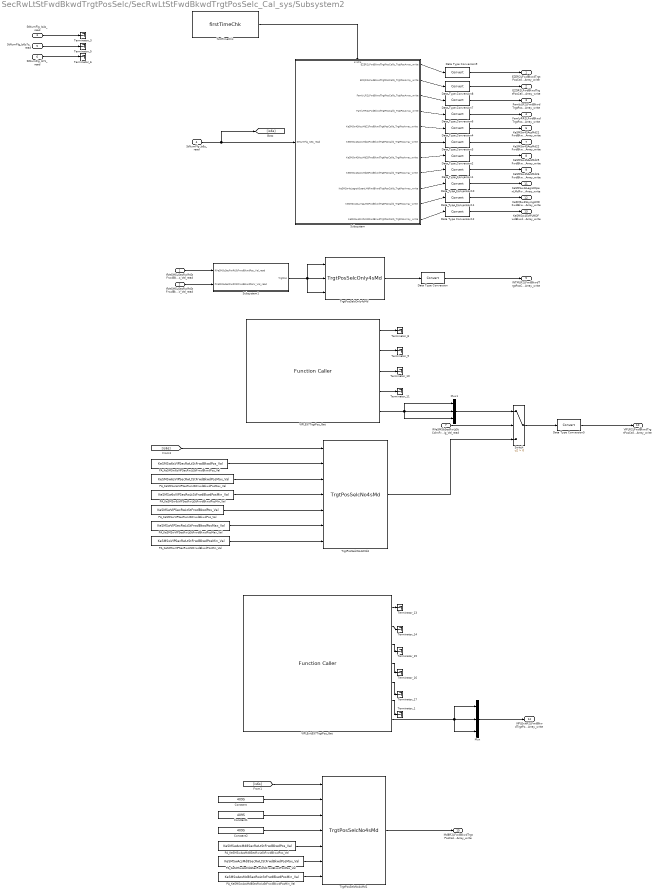
== system SecRwLtStFwdBkwdTrgtPosSelc/SecRwLtStFwdBkwdTrgtPosSelc_Cal_sys/Subsystem2 ==
  IfVeSMSuSecRwRtStFrwdBkwdPos_Val_read : Inport
  IfVeSMSuSecRwRtStFrwdBkwdPosV_Val_read : Inport  Port=2
  StNumFlg_Is4s_read : Inport  Port=3
  StNumFlg_Is6s_read : Inport  Port=4
  StNumFlg_Is6s7s_read : Inport  Port=5
  StNumFlg_Is7s_read : Inport  Port=6
  IfVeSMSbSecRwLtStCshnFrntUpwdDnwdMovConfig_Val_read : Inport  Port=7
  Constant : Constant  Value=4095  OutDataTypeStr=uint16
  Constant1 : Constant  Value=4095  OutDataTypeStr=uint16
  Constant2 : Constant  Value=4095  OutDataTypeStr=uint16
  Data Type Conversion{,1..12} (13 alike) : DataTypeConversion
  Mux : Mux  Inputs=3
  Mux1 : Mux  Inputs=3
  PA_KeSMSw6sVIPSecRwLtStFrwdBkwdPosMax_Val : Constant  Value=KeSMSw6sVIPSecRwLtStFrwdBkwdPosMax_Val
  PA_KeSMSw6sVIPSecRwLtStFrwdBkwdPosMin_Val : Constant  Value=KeSMSw6sVIPSecRwLtStFrwdBkwdPosMin_Val
  PA_KeSMSw6sVIPSecRwLtStFrwdBkwdPos_Val : Constant  Value=KeSMSw6sVIPSecRwLtStFrwdBkwdPos_Val
  PA_KeSMSwAcsMd8SecRwLtStFrwdBkwdPosMax_Val : Constant  Value=KeSMSwAcsMd8SecRwLtStFrwdBkwdPosMax_Val
  PA_KeSMSwAcsMd8SecRwLtStFrwdBkwdPosMin_Val : Constant  Value=KeSMSwAcsMd8SecRwLtStFrwdBkwdPosMin_Val
  PA_KeSMSwAcsMd8SecRwLtStFrwdBkwdPos_Val : Constant  Value=KeSMSwAcsMd8SecRwLtStFrwdBkwdPos_Val
  PA_KeSMSwVIPSecRwLtStFrwdBkwdPosMax_Val : Constant  Value=KeSMSwVIPSecRwLtStFrwdBkwdPosMax_Val
  PA_KeSMSwVIPSecRwLtStFrwdBkwdPosMin_Val : Constant  Value=KeSMSwVIPSecRwLtStFrwdBkwdPosMin_Val
  PA_KeSMSwVIPSecRwLtStFrwdBkwdPos_Val : Constant  Value=KeSMSwVIPSecRwLtStFrwdBkwdPos_Val
  Subsystem : Subsystem
  Subsystem1 : Subsystem
  Switch : Switch  Criteria=u2 > Threshold
  Terminator_{1,3,5..6,8..11,13..17} (13 alike) : Terminator
  TrgtPosSelcNo4sMd1 : TrgtPosSelcLib/TrgtPosSelcNo4sMd  SystemSampleTime=-1
  TrgtPosSelcNo4sMd4 : TrgtPosSelcLib/TrgtPosSelcNo4sMd  SystemSampleTime=-1
  TrgtPosSelcOnly4sMd : TrgtPosSelcLib/TrgtPosSelcOnly4sMd  SystemSampleTime=-1
  VIPL557TrgtPos_Get : FunctionCaller  FunctionPrototype=[SecRwLtStBkReclnTrgtPos,SecRwLtStZeroTrgtPos,SecRwLtStLgrstUpwdDnwdTrgtPos,SecRwLtStLgrstInwdOtwdTrgtPos,SecRwLtStFwdBkwdTrgtPos] = VIPL557TrgtPos_Get()  OutputArgumentSpecifications=uint16(1), uint16(1), uint16(1), uint16(1), uint16(1)
  VIPLExit557TrgtPos_Get : FunctionCaller  FunctionPrototype=[SecRwLtStBkReclnTrgtPos,SecRwLtStZeroTrgtPos,SecRwLtStLgrstUpwdDnwdTrgtPos,SecRwLtStLgrstInwdOtwdTrgtPos,ThdRwLtStBkReclnTrgtPos,ThdRwLtStFwdBkwdTrgtPos,SecRwLtStFwdBkwdTrgtPos] = VIPLExit557TrgtPos_Get()  OutputArgumentSpecifications=uint16(1), uint16(1), uint16(1), uint16(1), uint16(1), uint16(1), uint16(1)
  firstTimeChk : TrgtPosSelcLib/firstTimeChk  SystemSampleTime=-1
  EZER2LFwdBkwdTrgtPosCalib_TrgtPosArray_write : Outport
      settings: EnsureOutportIsVirtual=on
  EZQR2LFwdBkwdTrgtPosCalib_TrgtPosArray_write : Outport  Port=2
      settings: EnsureOutportIsVirtual=on
  FamlyLR2LFwdBkwdTrgtPosCalib_TrgtPosArray_write : Outport  Port=3
      settings: EnsureOutportIsVirtual=on
  FamlyRR2LFwdBkwdTrgtPosCalib_TrgtPosArray_write : Outport  Port=4
      settings: EnsureOutportIsVirtual=on
  INTMLR2LFwdBkwdTrgtPosCalib_TrgtPosArray_write : Outport  Port=5
      settings: EnsureOutportIsVirtual=on
  KeSMSw4SAcsMd21FwdBkwdTrgtPosCalib_TrgtPosArray_write : Outport  Port=6
      settings: EnsureOutportIsVirtual=on
  KeSMSw4SAcsMd22FwdBkwdTrgtPosCalib_TrgtPosArray_write : Outport  Port=7
      settings: EnsureOutportIsVirtual=on
  KeSMSw4SAcsMd25FwdBkwdTrgtPosCalib_TrgtPosArray_write : Outport  Port=8
      settings: EnsureOutportIsVirtual=on
  KeSMSw4SAcsMd26FwdBkwdTrgtPosCalib_TrgtPosArray_write : Outport  Port=9
      settings: EnsureOutportIsVirtual=on
  VIPLR2LFwdBkwdTrgtPosCalib_TrgtPosArray_write : Outport  Port=10
      settings: EnsureOutportIsVirtual=on
  KeSMSw4sLegrstOpenLMdFwdBkwdTrgtPosCalib_TrgtPosArray_write : Outport  Port=11
      settings: EnsureOutportIsVirtual=on
  KeSMSw4SLyingLMDFwdBkwdTrgtPosCalib_TrgtPosArray_write : Outport  Port=12
      settings: EnsureOutportIsVirtual=on
  KeSMSw4SVIPLMDFwdBkwdTrgtPosCalib_TrgtPosArray_write : Outport  Port=13
      settings: EnsureOutportIsVirtual=on
  VIPLExitR2LFwdBkwdTrgtPosCalib_TrgtPosArray_write : Outport  Port=14
      settings: EnsureOutportIsVirtual=on
  Md8R2LFwdBkwdTrgtPosCalib_TrgtPosArray_write : Outport  Port=15
      settings: EnsureOutportIsVirtual=on
  wires:
  Subsystem/1(EZER2LFwdBkwdTrgtPosCalib_TrgtPosArray_write) -> Data Type Conversion9/1
  StNumFlg_Is4s_read/1 -> Terminator_3/1
  Subsystem1/1(TrgtPos) -> TrgtPosSelcOnly4sMd/2, TrgtPosSelcOnly4sMd/1, TrgtPosSelcOnly4sMd/3
  IfVeSMSuSecRwRtStFrwdBkwdPos_Val_read/1 -> Subsystem1/1(IfVeSMSuSecRwRtStFrwdBkwdPos_Val_read)
  Subsystem/3(FamlyLR2LFwdBkwdTrgtPosCalib_TrgtPosArray_write) -> Data Type Conversion7/1
  StNumFlg_Is6s7s_read/1 -> Terminator_5/1
  StNumFlg_Is7s_read/1 -> Terminator_6/1
  Subsystem/4(FamlyRR2LFwdBkwdTrgtPosCalib_TrgtPosArray_write) -> Data Type Conversion6/1
  Switch/1 -> Data Type Conversion5/1
  StNumFlg_Is6s_read/1 -> [is6s], Subsystem/1(StNumFlg_Is6s_read)
  Subsystem/2(EZQR2LFwdBkwdTrgtPosCalib_TrgtPosArray_write) -> Data Type Conversion8/1
  firstTimeChk/1 -> Subsystem/Enable
  TrgtPosSelcOnly4sMd/1 -> Data Type Conversion/1
  IfVeSMSuSecRwRtStFrwdBkwdPosV_Val_read/1 -> Subsystem1/2(IfVeSMSuSecRwRtStFrwdBkwdPosV_Val_read)
  Subsystem/8(KeSMSw4SAcsMd26FwdBkwdTrgtPosCalib_TrgtPosArray_write) -> Data Type Conversion1/1
  Subsystem/7(KeSMSw4SAcsMd25FwdBkwdTrgtPosCalib_TrgtPosArray_write) -> Data Type Conversion2/1
  Subsystem/6(KeSMSw4SAcsMd22FwdBkwdTrgtPosCalib_TrgtPosArray_write) -> Data Type Conversion3/1
  Subsystem/5(KeSMSw4SAcsMd21FwdBkwdTrgtPosCalib_TrgtPosArray_write) -> Data Type Conversion4/1
  Data Type Conversion/1 -> INTMLR2LFwdBkwdTrgtPosCalib_TrgtPosArray_write/1
  Data Type Conversion1/1 -> KeSMSw4SAcsMd26FwdBkwdTrgtPosCalib_TrgtPosArray_write/1
  Data Type Conversion2/1 -> KeSMSw4SAcsMd25FwdBkwdTrgtPosCalib_TrgtPosArray_write/1
  Data Type Conversion3/1 -> KeSMSw4SAcsMd22FwdBkwdTrgtPosCalib_TrgtPosArray_write/1
  Data Type Conversion4/1 -> KeSMSw4SAcsMd21FwdBkwdTrgtPosCalib_TrgtPosArray_write/1
  Data Type Conversion5/1 -> VIPLR2LFwdBkwdTrgtPosCalib_TrgtPosArray_write/1
  Data Type Conversion6/1 -> FamlyRR2LFwdBkwdTrgtPosCalib_TrgtPosArray_write/1
  Data Type Conversion7/1 -> FamlyLR2LFwdBkwdTrgtPosCalib_TrgtPosArray_write/1
  Data Type Conversion8/1 -> EZQR2LFwdBkwdTrgtPosCalib_TrgtPosArray_write/1
  Data Type Conversion9/1 -> EZER2LFwdBkwdTrgtPosCalib_TrgtPosArray_write/1
  Data Type Conversion12/1 -> KeSMSw4SVIPLMDFwdBkwdTrgtPosCalib_TrgtPosArray_write/1
  Data Type Conversion10/1 -> KeSMSw4sLegrstOpenLMdFwdBkwdTrgtPosCalib_TrgtPosArray_write/1
  Data Type Conversion11/1 -> KeSMSw4SLyingLMDFwdBkwdTrgtPosCalib_TrgtPosArray_write/1
  Subsystem/9(KeSMSw4sLegrstOpenLMdFwdBkwdTrgtPosCalib_TrgtPosArray_write) -> Data Type Conversion10/1
  Subsystem/10(KeSMSw4SLyingLMDFwdBkwdTrgtPosCalib_TrgtPosArray_write) -> Data Type Conversion11/1
  Subsystem/11(KeSMSw4SVIPLMDFwdBkwdTrgtPosCalib_TrgtPosArray_write) -> Data Type Conversion12/1
  IfVeSMSbSecRwLtStCshnFrntUpwdDnwdMovConfig_Val_read/1 -> Switch/2
  [is6s] -> TrgtPosSelcNo4sMd4/1
  PA_KeSMSwVIPSecRwLtStFrwdBkwdPos_Val/1 -> TrgtPosSelcNo4sMd4/5
  PA_KeSMSwVIPSecRwLtStFrwdBkwdPosMax_Val/1 -> TrgtPosSelcNo4sMd4/6
  PA_KeSMSw6sVIPSecRwLtStFrwdBkwdPosMin_Val/1 -> TrgtPosSelcNo4sMd4/4
  PA_KeSMSw6sVIPSecRwLtStFrwdBkwdPos_Val/1 -> TrgtPosSelcNo4sMd4/2
  PA_KeSMSwVIPSecRwLtStFrwdBkwdPosMin_Val/1 -> TrgtPosSelcNo4sMd4/7
  PA_KeSMSw6sVIPSecRwLtStFrwdBkwdPosMax_Val/1 -> TrgtPosSelcNo4sMd4/3
  TrgtPosSelcNo4sMd4/1 -> Switch/3
  VIPL557TrgtPos_Get/1 -> Terminator_8/1
  VIPL557TrgtPos_Get/2 -> Terminator_9/1
  VIPL557TrgtPos_Get/3 -> Terminator_10/1
  VIPL557TrgtPos_Get/4 -> Terminator_11/1
  VIPLExit557TrgtPos_Get/1 -> Terminator_13/1
  VIPLExit557TrgtPos_Get/2 -> Terminator_14/1
  VIPLExit557TrgtPos_Get/3 -> Terminator_15/1
  VIPLExit557TrgtPos_Get/4 -> Terminator_16/1
  VIPLExit557TrgtPos_Get/5 -> Terminator_17/1
  Mux/1 -> VIPLExitR2LFwdBkwdTrgtPosCalib_TrgtPosArray_write/1
  Mux1/1 -> Switch/1
  VIPL557TrgtPos_Get/5 -> Mux1/3, Mux1/2, Mux1/1
  VIPLExit557TrgtPos_Get/7 -> Mux/3, Mux/1, Mux/2
  VIPLExit557TrgtPos_Get/6 -> Terminator_1/1
  [is6s] -> TrgtPosSelcNo4sMd1/1
  PA_KeSMSwAcsMd8SecRwLtStFrwdBkwdPos_Val/1 -> TrgtPosSelcNo4sMd1/5
  PA_KeSMSwAcsMd8SecRwLtStFrwdBkwdPosMax_Val/1 -> TrgtPosSelcNo4sMd1/6
  PA_KeSMSwAcsMd8SecRwLtStFrwdBkwdPosMin_Val/1 -> TrgtPosSelcNo4sMd1/7
  TrgtPosSelcNo4sMd1/1 -> Md8R2LFwdBkwdTrgtPosCalib_TrgtPosArray_write/1
  Constant/1 -> TrgtPosSelcNo4sMd1/2
  Constant1/1 -> TrgtPosSelcNo4sMd1/3
  Constant2/1 -> TrgtPosSelcNo4sMd1/4

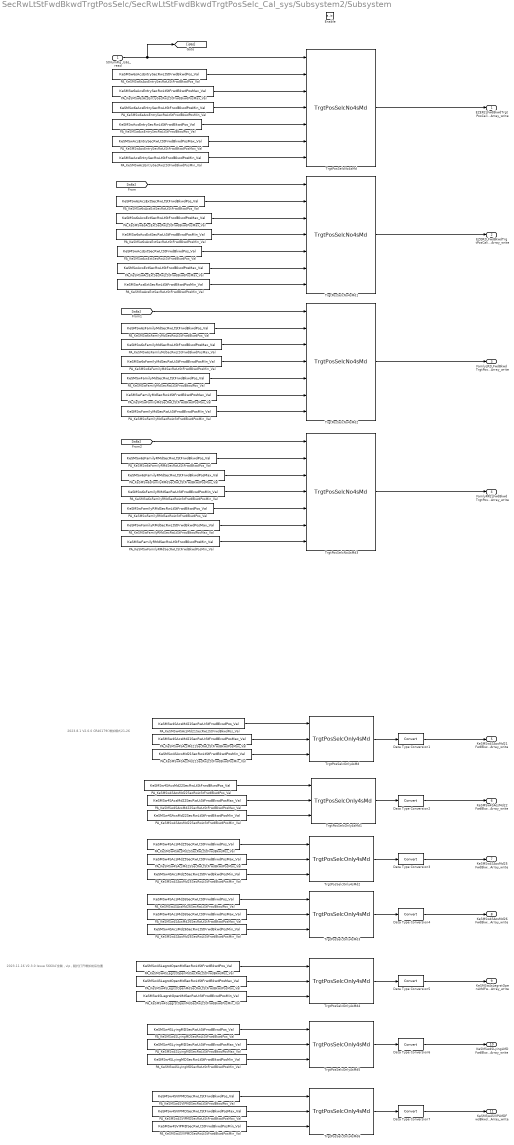
== system SecRwLtStFwdBkwdTrgtPosSelc/SecRwLtStFwdBkwdTrgtPosSelc_Cal_sys/Subsystem2/Subsystem ==
  note: 2023.11.16 V2.3.0 Issue 566045 全躺，vip，腿托打开增加前后位置
  note: 2023.8.1 V2.0.0 CR401790 增加模式21-26
  StNumFlg_Is6s_read : Inport
  Enable : EnablePort
  Data Type Conversion{1..7} (7 alike) : DataTypeConversion
  PA_KeSMSw4SAcsMd21SecRwLtStFrwdBkwdPosMax_Val : Constant  Value=KeSMSw4SAcsMd21SecRwLtStFrwdBkwdPosMax_Val
  PA_KeSMSw4SAcsMd21SecRwLtStFrwdBkwdPosMin_Val : Constant  Value=KeSMSw4SAcsMd21SecRwLtStFrwdBkwdPosMin_Val
  PA_KeSMSw4SAcsMd21SecRwLtStFrwdBkwdPos_Val : Constant  Value=KeSMSw4SAcsMd21SecRwLtStFrwdBkwdPos_Val
  PA_KeSMSw4SAcsMd22SecRwLtStFrwdBkwdPosMax_Val : Constant  Value=KeSMSw4SAcsMd22SecRwLtStFrwdBkwdPosMax_Val
  PA_KeSMSw4SAcsMd22SecRwLtStFrwdBkwdPosMin_Val : Constant  Value=KeSMSw4SAcsMd22SecRwLtStFrwdBkwdPosMin_Val
  PA_KeSMSw4SAcsMd22SecRwLtStFrwdBkwdPos_Val : Constant  Value=KeSMSw4SAcsMd22SecRwLtStFrwdBkwdPos_Val
  PA_KeSMSw4SAcsMd25SecRwLtStFrwdBkwdPosMax_Val : Constant  Value=KeSMSw4SAcsMd25SecRwLtStFrwdBkwdPosMax_Val
  PA_KeSMSw4SAcsMd25SecRwLtStFrwdBkwdPosMin_Val : Constant  Value=KeSMSw4SAcsMd25SecRwLtStFrwdBkwdPosMin_Val
  PA_KeSMSw4SAcsMd25SecRwLtStFrwdBkwdPos_Val : Constant  Value=KeSMSw4SAcsMd25SecRwLtStFrwdBkwdPos_Val
  PA_KeSMSw4SAcsMd26SecRwLtStFrwdBkwdPosMax_Val : Constant  Value=KeSMSw4SAcsMd26SecRwLtStFrwdBkwdPosMax_Val
  PA_KeSMSw4SAcsMd26SecRwLtStFrwdBkwdPosMin_Val : Constant  Value=KeSMSw4SAcsMd26SecRwLtStFrwdBkwdPosMin_Val
  PA_KeSMSw4SAcsMd26SecRwLtStFrwdBkwdPos_Val : Constant  Value=KeSMSw4SAcsMd26SecRwLtStFrwdBkwdPos_Val
  PA_KeSMSw4SLegrstOpenMdSecRwLtStFrwdBkwdPosMax_Val : Constant  Value=KeSMSw4SLegrstOpenMdSecRwLtStFrwdBkwdPosMax_Val
  PA_KeSMSw4SLegrstOpenMdSecRwLtStFrwdBkwdPosMin_Val : Constant  Value=KeSMSw4SLegrstOpenMdSecRwLtStFrwdBkwdPosMin_Val
  PA_KeSMSw4SLegrstOpenMdSecRwLtStFrwdBkwdPos_Val : Constant  Value=KeSMSw4SLegrstOpenMdSecRwLtStFrwdBkwdPos_Val
  PA_KeSMSw4SLyingMDSecRwLtStFrwdBkwdPosMax_Val : Constant  Value=KeSMSw4SLyingMDSecRwLtStFrwdBkwdPosMax_Val
  PA_KeSMSw4SLyingMDSecRwLtStFrwdBkwdPosMin_Val : Constant  Value=KeSMSw4SLyingMDSecRwLtStFrwdBkwdPosMin_Val
  PA_KeSMSw4SLyingMDSecRwLtStFrwdBkwdPos_Val : Constant  Value=KeSMSw4SLyingMDSecRwLtStFrwdBkwdPos_Val
  PA_KeSMSw4SVIPMDSecRwLtStFrwdBkwdPosMax_Val : Constant  Value=KeSMSw4SVIPMDSecRwLtStFrwdBkwdPosMax_Val
  PA_KeSMSw4SVIPMDSecRwLtStFrwdBkwdPosMin_Val : Constant  Value=KeSMSw4SVIPMDSecRwLtStFrwdBkwdPosMin_Val
  PA_KeSMSw4SVIPMDSecRwLtStFrwdBkwdPos_Val : Constant  Value=KeSMSw4SVIPMDSecRwLtStFrwdBkwdPos_Val
  PA_KeSMSw6sAcsEntrySecRwLtStFrwdBkwdPosMax_Val : Constant  Value=KeSMSw6sAcsEntrySecRwLtStFrwdBkwdPosMax_Val
  PA_KeSMSw6sAcsEntrySecRwLtStFrwdBkwdPosMin_Val : Constant  Value=KeSMSw6sAcsEntrySecRwLtStFrwdBkwdPosMin_Val
  PA_KeSMSw6sAcsEntrySecRwLtStFrwdBkwdPos_Val : Constant  Value=KeSMSw6sAcsEntrySecRwLtStFrwdBkwdPos_Val
  PA_KeSMSw6sAcsExtSecRwLtStFrwdBkwdPosMax_Val : Constant  Value=KeSMSw6sAcsExtSecRwLtStFrwdBkwdPosMax_Val
  PA_KeSMSw6sAcsExtSecRwLtStFrwdBkwdPosMin_Val : Constant  Value=KeSMSw6sAcsExtSecRwLtStFrwdBkwdPosMin_Val
  PA_KeSMSw6sAcsExtSecRwLtStFrwdBkwdPos_Val : Constant  Value=KeSMSw6sAcsExtSecRwLtStFrwdBkwdPos_Val
  PA_KeSMSw6sFamilyMdSecRwLtStFrwdBkwdPosMax_Val : Constant  Value=KeSMSw6sFamilyMdSecRwLtStFrwdBkwdPosMax_Val
  PA_KeSMSw6sFamilyMdSecRwLtStFrwdBkwdPosMin_Val : Constant  Value=KeSMSw6sFamilyMdSecRwLtStFrwdBkwdPosMin_Val
  PA_KeSMSw6sFamilyMdSecRwLtStFrwdBkwdPos_Val : Constant  Value=KeSMSw6sFamilyMdSecRwLtStFrwdBkwdPos_Val
  PA_KeSMSw6sFamilyRMdSecRwLtStFrwdBkwdPosMax_Val : Constant  Value=KeSMSw6sFamilyRMdSecRwLtStFrwdBkwdPosMax_Val
  PA_KeSMSw6sFamilyRMdSecRwLtStFrwdBkwdPosMin_Val : Constant  Value=KeSMSw6sFamilyRMdSecRwLtStFrwdBkwdPosMin_Val
  PA_KeSMSw6sFamilyRMdSecRwLtStFrwdBkwdPos_Val : Constant  Value=KeSMSw6sFamilyRMdSecRwLtStFrwdBkwdPos_Val
  PA_KeSMSwAcsEntrySecRwLtStFrwdBkwdPosMax_Val : Constant  Value=KeSMSwAcsEntrySecRwLtStFrwdBkwdPosMax_Val
  PA_KeSMSwAcsEntrySecRwLtStFrwdBkwdPosMin_Val : Constant  Value=KeSMSwAcsEntrySecRwLtStFrwdBkwdPosMin_Val
  PA_KeSMSwAcsEntrySecRwLtStFrwdBkwdPos_Val : Constant  Value=KeSMSwAcsEntrySecRwLtStFrwdBkwdPos_Val
  PA_KeSMSwAcsExtSecRwLtStFrwdBkwdPosMax_Val : Constant  Value=KeSMSwAcsExtSecRwLtStFrwdBkwdPosMax_Val
  PA_KeSMSwAcsExtSecRwLtStFrwdBkwdPosMin_Val : Constant  Value=KeSMSwAcsExtSecRwLtStFrwdBkwdPosMin_Val
  PA_KeSMSwAcsExtSecRwLtStFrwdBkwdPos_Val : Constant  Value=KeSMSwAcsExtSecRwLtStFrwdBkwdPos_Val
  PA_KeSMSwFamilyMdSecRwLtStFrwdBkwdPosMax_Val : Constant  Value=KeSMSwFamilyMdSecRwLtStFrwdBkwdPosMax_Val
  PA_KeSMSwFamilyMdSecRwLtStFrwdBkwdPosMin_Val : Constant  Value=KeSMSwFamilyMdSecRwLtStFrwdBkwdPosMin_Val
  PA_KeSMSwFamilyMdSecRwLtStFrwdBkwdPos_Val : Constant  Value=KeSMSwFamilyMdSecRwLtStFrwdBkwdPos_Val
  PA_KeSMSwFamilyRMdSecRwLtStFrwdBkwdPosMax_Val : Constant  Value=KeSMSwFamilyRMdSecRwLtStFrwdBkwdPosMax_Val
  PA_KeSMSwFamilyRMdSecRwLtStFrwdBkwdPosMin_Val : Constant  Value=KeSMSwFamilyRMdSecRwLtStFrwdBkwdPosMin_Val
  PA_KeSMSwFamilyRMdSecRwLtStFrwdBkwdPos_Val : Constant  Value=KeSMSwFamilyRMdSecRwLtStFrwdBkwdPos_Val
  TrgtPosSelcNo4sMd{,1..3} (4 alike) : TrgtPosSelcLib/TrgtPosSelcNo4sMd  SystemSampleTime=-1
  TrgtPosSelcOnly4sMd{,1..6} (7 alike) : TrgtPosSelcLib/TrgtPosSelcOnly4sMd  SystemSampleTime=-1
  EZER2LFwdBkwdTrgtPosCalib_TrgtPosArray_write : Outport
      settings: EnsureOutportIsVirtual=on
  EZQR2LFwdBkwdTrgtPosCalib_TrgtPosArray_write : Outport  Port=2
      settings: EnsureOutportIsVirtual=on
  FamlyLR2LFwdBkwdTrgtPosCalib_TrgtPosArray_write : Outport  Port=3
      settings: EnsureOutportIsVirtual=on
  FamlyRR2LFwdBkwdTrgtPosCalib_TrgtPosArray_write : Outport  Port=4
      settings: EnsureOutportIsVirtual=on
  KeSMSw4SAcsMd21FwdBkwdTrgtPosCalib_TrgtPosArray_write : Outport  Port=5
      settings: EnsureOutportIsVirtual=on
  KeSMSw4SAcsMd22FwdBkwdTrgtPosCalib_TrgtPosArray_write : Outport  Port=6
      settings: EnsureOutportIsVirtual=on
  KeSMSw4SAcsMd25FwdBkwdTrgtPosCalib_TrgtPosArray_write : Outport  Port=7
      settings: EnsureOutportIsVirtual=on
  KeSMSw4SAcsMd26FwdBkwdTrgtPosCalib_TrgtPosArray_write : Outport  Port=8
      settings: EnsureOutportIsVirtual=on
  KeSMSw4sLegrstOpenLMdFwdBkwdTrgtPosCalib_TrgtPosArray_write : Outport  Port=9
      settings: EnsureOutportIsVirtual=on
  KeSMSw4SLyingLMDFwdBkwdTrgtPosCalib_TrgtPosArray_write : Outport  Port=10
      settings: EnsureOutportIsVirtual=on
  KeSMSw4SVIPLMDFwdBkwdTrgtPosCalib_TrgtPosArray_write : Outport  Port=11
      settings: EnsureOutportIsVirtual=on
  wires:
  TrgtPosSelcNo4sMd1/1 -> EZQR2LFwdBkwdTrgtPosCalib_TrgtPosArray_write/1
  TrgtPosSelcNo4sMd3/1 -> FamlyRR2LFwdBkwdTrgtPosCalib_TrgtPosArray_write/1
  TrgtPosSelcNo4sMd/1 -> EZER2LFwdBkwdTrgtPosCalib_TrgtPosArray_write/1
  TrgtPosSelcNo4sMd2/1 -> FamlyLR2LFwdBkwdTrgtPosCalib_TrgtPosArray_write/1
  StNumFlg_Is6s_read/1 -> [is6s], TrgtPosSelcNo4sMd/1
  PA_KeSMSw6sAcsEntrySecRwLtStFrwdBkwdPos_Val/1 -> TrgtPosSelcNo4sMd/2
  PA_KeSMSw6sAcsEntrySecRwLtStFrwdBkwdPosMax_Val/1 -> TrgtPosSelcNo4sMd/3
  PA_KeSMSw6sAcsEntrySecRwLtStFrwdBkwdPosMin_Val/1 -> TrgtPosSelcNo4sMd/4
  PA_KeSMSw6sAcsExtSecRwLtStFrwdBkwdPosMin_Val/1 -> TrgtPosSelcNo4sMd1/4
  PA_KeSMSw6sAcsExtSecRwLtStFrwdBkwdPosMax_Val/1 -> TrgtPosSelcNo4sMd1/3
  PA_KeSMSw6sAcsExtSecRwLtStFrwdBkwdPos_Val/1 -> TrgtPosSelcNo4sMd1/2
  PA_KeSMSw6sFamilyMdSecRwLtStFrwdBkwdPos_Val/1 -> TrgtPosSelcNo4sMd2/2
  PA_KeSMSw6sFamilyMdSecRwLtStFrwdBkwdPosMax_Val/1 -> TrgtPosSelcNo4sMd2/3
  PA_KeSMSw6sFamilyMdSecRwLtStFrwdBkwdPosMin_Val/1 -> TrgtPosSelcNo4sMd2/4
  PA_KeSMSw6sFamilyRMdSecRwLtStFrwdBkwdPosMin_Val/1 -> TrgtPosSelcNo4sMd3/4
  PA_KeSMSw6sFamilyRMdSecRwLtStFrwdBkwdPosMax_Val/1 -> TrgtPosSelcNo4sMd3/3
  PA_KeSMSw6sFamilyRMdSecRwLtStFrwdBkwdPos_Val/1 -> TrgtPosSelcNo4sMd3/2
  PA_KeSMSwAcsEntrySecRwLtStFrwdBkwdPos_Val/1 -> TrgtPosSelcNo4sMd/5
  PA_KeSMSwAcsEntrySecRwLtStFrwdBkwdPosMax_Val/1 -> TrgtPosSelcNo4sMd/6
  PA_KeSMSwAcsEntrySecRwLtStFrwdBkwdPosMin_Val/1 -> TrgtPosSelcNo4sMd/7
  PA_KeSMSwAcsExtSecRwLtStFrwdBkwdPos_Val/1 -> TrgtPosSelcNo4sMd1/5
  PA_KeSMSwAcsExtSecRwLtStFrwdBkwdPosMax_Val/1 -> TrgtPosSelcNo4sMd1/6
  PA_KeSMSwAcsExtSecRwLtStFrwdBkwdPosMin_Val/1 -> TrgtPosSelcNo4sMd1/7
  PA_KeSMSwFamilyMdSecRwLtStFrwdBkwdPosMin_Val/1 -> TrgtPosSelcNo4sMd2/7
  PA_KeSMSwFamilyMdSecRwLtStFrwdBkwdPosMax_Val/1 -> TrgtPosSelcNo4sMd2/6
  PA_KeSMSwFamilyMdSecRwLtStFrwdBkwdPos_Val/1 -> TrgtPosSelcNo4sMd2/5
  PA_KeSMSwFamilyRMdSecRwLtStFrwdBkwdPos_Val/1 -> TrgtPosSelcNo4sMd3/5
  PA_KeSMSwFamilyRMdSecRwLtStFrwdBkwdPosMax_Val/1 -> TrgtPosSelcNo4sMd3/6
  PA_KeSMSwFamilyRMdSecRwLtStFrwdBkwdPosMin_Val/1 -> TrgtPosSelcNo4sMd3/7
  [is6s] -> TrgtPosSelcNo4sMd1/1
  [is6s] -> TrgtPosSelcNo4sMd2/1
  [is6s] -> TrgtPosSelcNo4sMd3/1
  TrgtPosSelcOnly4sMd/1 -> Data Type Conversion1/1
  TrgtPosSelcOnly4sMd3/1 -> Data Type Conversion4/1
  TrgtPosSelcOnly4sMd2/1 -> Data Type Conversion3/1
  TrgtPosSelcOnly4sMd1/1 -> Data Type Conversion2/1
  PA_KeSMSw4SAcsMd26SecRwLtStFrwdBkwdPosMax_Val/1 -> TrgtPosSelcOnly4sMd3/2
  PA_KeSMSw4SAcsMd26SecRwLtStFrwdBkwdPosMin_Val/1 -> TrgtPosSelcOnly4sMd3/3
  PA_KeSMSw4SAcsMd26SecRwLtStFrwdBkwdPos_Val/1 -> TrgtPosSelcOnly4sMd3/1
  PA_KeSMSw4SAcsMd25SecRwLtStFrwdBkwdPosMax_Val/1 -> TrgtPosSelcOnly4sMd2/2
  PA_KeSMSw4SAcsMd25SecRwLtStFrwdBkwdPosMin_Val/1 -> TrgtPosSelcOnly4sMd2/3
  PA_KeSMSw4SAcsMd25SecRwLtStFrwdBkwdPos_Val/1 -> TrgtPosSelcOnly4sMd2/1
  PA_KeSMSw4SAcsMd22SecRwLtStFrwdBkwdPosMax_Val/1 -> TrgtPosSelcOnly4sMd1/2
  PA_KeSMSw4SAcsMd22SecRwLtStFrwdBkwdPosMin_Val/1 -> TrgtPosSelcOnly4sMd1/3
  PA_KeSMSw4SAcsMd22SecRwLtStFrwdBkwdPos_Val/1 -> TrgtPosSelcOnly4sMd1/1
  PA_KeSMSw4SAcsMd21SecRwLtStFrwdBkwdPosMax_Val/1 -> TrgtPosSelcOnly4sMd/2
  PA_KeSMSw4SAcsMd21SecRwLtStFrwdBkwdPosMin_Val/1 -> TrgtPosSelcOnly4sMd/3
  PA_KeSMSw4SAcsMd21SecRwLtStFrwdBkwdPos_Val/1 -> TrgtPosSelcOnly4sMd/1
  Data Type Conversion1/1 -> KeSMSw4SAcsMd21FwdBkwdTrgtPosCalib_TrgtPosArray_write/1
  Data Type Conversion2/1 -> KeSMSw4SAcsMd22FwdBkwdTrgtPosCalib_TrgtPosArray_write/1
  Data Type Conversion3/1 -> KeSMSw4SAcsMd25FwdBkwdTrgtPosCalib_TrgtPosArray_write/1
  Data Type Conversion4/1 -> KeSMSw4SAcsMd26FwdBkwdTrgtPosCalib_TrgtPosArray_write/1
  PA_KeSMSw4SLegrstOpenMdSecRwLtStFrwdBkwdPos_Val/1 -> TrgtPosSelcOnly4sMd4/1
  PA_KeSMSw4SLegrstOpenMdSecRwLtStFrwdBkwdPosMin_Val/1 -> TrgtPosSelcOnly4sMd4/3
  PA_KeSMSw4SLegrstOpenMdSecRwLtStFrwdBkwdPosMax_Val/1 -> TrgtPosSelcOnly4sMd4/2
  TrgtPosSelcOnly4sMd4/1 -> Data Type Conversion5/1
  TrgtPosSelcOnly4sMd5/1 -> Data Type Conversion6/1
  PA_KeSMSw4SLyingMDSecRwLtStFrwdBkwdPosMax_Val/1 -> TrgtPosSelcOnly4sMd5/2
  PA_KeSMSw4SLyingMDSecRwLtStFrwdBkwdPosMin_Val/1 -> TrgtPosSelcOnly4sMd5/3
  PA_KeSMSw4SLyingMDSecRwLtStFrwdBkwdPos_Val/1 -> TrgtPosSelcOnly4sMd5/1
  PA_KeSMSw4SVIPMDSecRwLtStFrwdBkwdPos_Val/1 -> TrgtPosSelcOnly4sMd6/1
  PA_KeSMSw4SVIPMDSecRwLtStFrwdBkwdPosMin_Val/1 -> TrgtPosSelcOnly4sMd6/3
  PA_KeSMSw4SVIPMDSecRwLtStFrwdBkwdPosMax_Val/1 -> TrgtPosSelcOnly4sMd6/2
  TrgtPosSelcOnly4sMd6/1 -> Data Type Conversion7/1
  Data Type Conversion7/1 -> KeSMSw4SVIPLMDFwdBkwdTrgtPosCalib_TrgtPosArray_write/1
  Data Type Conversion5/1 -> KeSMSw4sLegrstOpenLMdFwdBkwdTrgtPosCalib_TrgtPosArray_write/1
  Data Type Conversion6/1 -> KeSMSw4SLyingLMDFwdBkwdTrgtPosCalib_TrgtPosArray_write/1

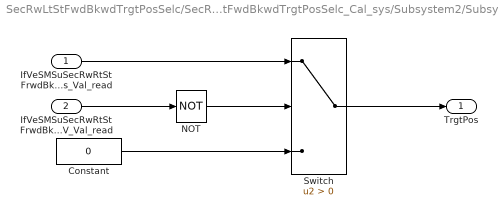
== system SecRwLtStFwdBkwdTrgtPosSelc/SecRwLtStFwdBkwdTrgtPosSelc_Cal_sys/Subsystem2/Subsystem1 ==
  IfVeSMSuSecRwRtStFrwdBkwdPos_Val_read : Inport
  IfVeSMSuSecRwRtStFrwdBkwdPosV_Val_read : Inport  Port=2
  Constant : Constant  Value=0  OutDataTypeStr=uint16
  NOT : Logic  Operator=NOT  AllPortsSameDT=off  OutDataTypeStr=boolean
  Switch : Switch  Criteria=u2 > Threshold
  TrgtPos : Outport
  wires:
  IfVeSMSuSecRwRtStFrwdBkwdPosV_Val_read/1 -> NOT/1
  Constant/1 -> Switch/3
  IfVeSMSuSecRwRtStFrwdBkwdPos_Val_read/1 -> Switch/1
  NOT/1 -> Switch/2
  Switch/1 -> TrgtPos/1
